simulink library "netZeroSpoolingControllerEllipsePath"  (R2020a)
settings: Solver=VariableStepAuto  StartTime=0.0  StopTime=10.0  RelTol=1e-3
undefined symbols (not defined in the file or in its folder): fltCtrl
libraries: runningAvg_ul x2, simulink x2, dspsigops x1
settings Model: Creator=jcreed2  LastModifiedBy=Josh Gaming
settings DataIOCC: ReturnWorkspaceOutputs=off
settings DebuggingCC: ArithmeticOperatorsInVariantConditions=warning
settings SFSimCC: CustomCodeUndefinedFunction=UseInterfaceOnly

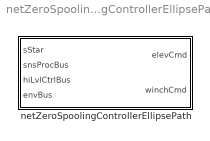
== system netZeroSpoolingControllerEllipsePath ==
  netZeroSpoolingControllerEllipsePath : Subsystem  mask{reelInDefl=23, reelOutDefl=0, sigmaVecInit=0, firstSpoolLap=fltCtrl.firstSpoolLap.Value}
      mask prompts: reelInDefl "Reel In Elevator Deflection [deg]"; reelOutDefl "Reel Out Elevator Deflection [deg]"; sigmaVecInit "Init Spooling Param Vec"; firstSpoolLap "First Lap to Start Spooling"

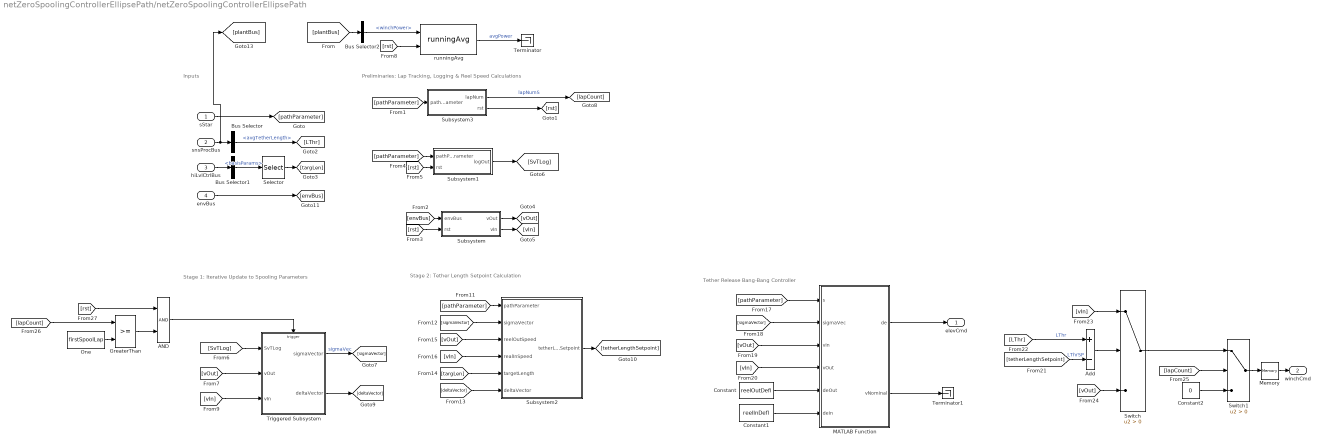
== system netZeroSpoolingControllerEllipsePath/netZeroSpoolingControllerEllipsePath ==
  note: Inputs
  note: Preliminaries: Lap Tracking, Logging & Reel Speed Calculations
  note: Stage 1: Iterative Update to Spooling Parameters
  note: Stage 2: Tether Length Setpoint Calculation
  note: Tether Release Bang-Bang Controller
  "sStar " : Inport
  snsProcBus : Inport  Port=2  OutDataTypeStr=Bus: sensorsProcessingBus
  hiLvlCtrlBus : Inport  Port=3  OutDataTypeStr=Bus: hiLvlCtrlBus
  envBus : Inport  Port=4  OutDataTypeStr=Bus: envBus
  AND : Logic  AllPortsSameDT=off  OutDataTypeStr=boolean
  Add : Sum  Inputs=+-
  Bus Selector : BusSelector  OutputSignals=avgTetherLength
  Bus Selector1 : BusSelector  OutputSignals=basisParams
  Bus Selector2 : BusSelector  OutputSignals=winchPower
  Constant : Constant  Value=reelOutDefl
  Constant1 : Constant  Value=reelInDefl
  Constant2 : Constant  Value=0
  GreaterThan : RelationalOperator  OutDataTypeStr=boolean  RndMeth=Simplest
  MATLAB Function : MATLAB Function  TreatAsAtomicUnit=on
  Memory : Memory
  One : Constant  Value=firstSpoolLap  OutDataTypeStr=Inherit: Inherit via back propagation
  Selector : Selector  InputPortWidth=5  IndexOptions=Index vector (dialog)  Indices=5  OutputSizes=1
  Subsystem : Subsystem
  Subsystem1 : Subsystem
  Subsystem2 : Subsystem
  Subsystem3 : Subsystem
  Switch : Switch  Criteria=u2 > Threshold
  Switch1 : Switch  Criteria=u2 > Threshold
  Terminator : Terminator
  Terminator1 : Terminator
  Triggered Subsystem : Subsystem  TreatAsAtomicUnit=on
  runningAvg : runningAvg_ul/runningAvg  SystemSampleTime=-1  Latency=0  AutoFrameSizeCalculation=off
  "elevCmd " : Outport  VectorParamsAs1DForOutWhenUnconnected=off
  winchCmd : Outport  Port=2  VectorParamsAs1DForOutWhenUnconnected=off
  wires:
  Switch/1 -> Switch1/1
  Constant/1 -> MATLAB Function/5(deOut)
  [rst] -> runningAvg/2
  [sigmaVector] -> MATLAB Function/2(sigmaVec)
  [lapCount] -> Switch1/2
  [vIn] -> Subsystem2/4(realInSpeed)
  runningAvg/1 -> Terminator/1  "avgPower"
  [rst] -> Subsystem1/2(rst)
  [SvTLog] -> Triggered Subsystem/1(SvTLog)
  "sStar "/1 -> [pathParameter]
  envBus/1 -> [envBus]
  Bus Selector1/1 -> Selector/1  "<basisParams>"
  [LThr] -> Add/1  "LThr"
  [pathParameter] -> Subsystem3/1(pathParameter)
  Bus Selector/1 -> [LThr]  "<avgTetherLength>"
  Add/1 -> Switch/2
  MATLAB Function/1(de) -> "elevCmd "/1
  Subsystem3/1(lapNum) -> [lapCount]  "lapNumS"
  [tetherLengthSetpoint] -> Add/2  "LThrSP"
  Constant1/1 -> MATLAB Function/6(deIn)
  Subsystem/2(vIn) -> [vIn]
  Constant2/1 -> Switch1/3
  [vOut] -> MATLAB Function/3(vIn)
  snsProcBus/1 -> [plantBus], Bus Selector/1
  Selector/1 -> [targLen]
  hiLvlCtrlBus/1 -> Bus Selector1/1
  [rst] -> Subsystem/2(rst)
  [vOut] -> Triggered Subsystem/2(vOut)
  Subsystem/1(vOut) -> [vOut]
  Triggered Subsystem/1("sigmaVector ") -> [sigmaVector]  "sigmaVec"
  [sigmaVector] -> Subsystem2/2(sigmaVector)
  [vIn] -> MATLAB Function/4(vOut)
  [deltaVector] -> Subsystem2/6(deltaVector)
  Subsystem3/2(rst) -> [rst]
  MATLAB Function/2(vNominal) -> Terminator1/1
  [vOut] -> Subsystem2/3(reelOutSpeed)
  [vIn] -> Switch/1
  [vIn] -> Triggered Subsystem/3(vIn)
  [pathParameter] -> MATLAB Function/1(s)
  Switch1/1 -> Memory/1
  [pathParameter] -> Subsystem2/1(pathParameter)
  [plantBus] -> Bus Selector2/1
  [targLen] -> Subsystem2/5(targetLength)
  [vOut] -> Switch/3
  Bus Selector2/1 -> runningAvg/1  "<winchPower>"
  [pathParameter] -> Subsystem1/1(pathParameter)
  [envBus] -> Subsystem/1(envBus)
  Triggered Subsystem/2(deltaVector) -> [deltaVector]
  Subsystem1/1(logOut) -> [SvTLog]
  GreaterThan/1 -> AND/2
  One/1 -> GreaterThan/2
  AND/1 -> Triggered Subsystem/Trigger
  [rst] -> AND/1
  [lapCount] -> GreaterThan/1
  Subsystem2/1(tetherLengthSetpoint) -> [tetherLengthSetpoint]
  Memory/1 -> winchCmd/1

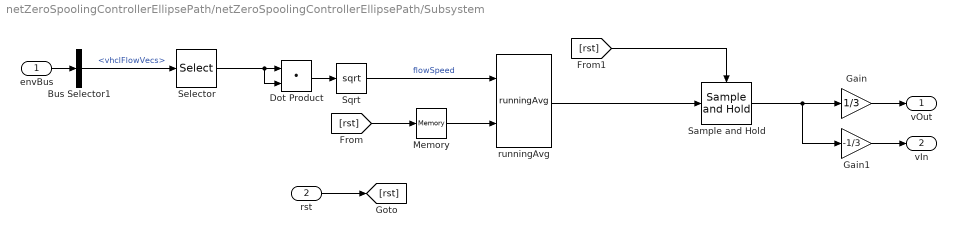
== system netZeroSpoolingControllerEllipsePath/netZeroSpoolingControllerEllipsePath/Subsystem ==
  envBus : Inport
  rst : Inport  Port=2
  Bus Selector1 : BusSelector  OutputSignals=vhclFlowVecs
  Dot Product : DotProduct  InputSameDT=on  OutDataTypeStr=Inherit: Inherit via internal rule
  Gain : Gain  Gain=1/3
  Gain1 : Gain  Gain=-1/3
  Memory : Memory
  Sample and Hold : dspsigops/Sample and Hold  trig=Rising edge  initCond=0  latchinput=off
  Selector : Selector  NumberOfDimensions=2  InputPortWidth=3  IndexOptions=Select all,Index vector (dialog)  Indices=[1 3],5  OutputSizes=1,1
  Sqrt : Sqrt  SaturateOnIntegerOverflow=on
  runningAvg : runningAvg_ul/runningAvg  SystemSampleTime=-1  Latency=0  AutoFrameSizeCalculation=off
  vOut : Outport  VectorParamsAs1DForOutWhenUnconnected=off
  vIn : Outport  Port=2  VectorParamsAs1DForOutWhenUnconnected=off
  wires:
  Dot Product/1 -> Sqrt/1
  Sample and Hold/1 -> Gain/1, Gain1/1
  Selector/1 -> Dot Product/1, Dot Product/2
  Sqrt/1 -> runningAvg/1  "flowSpeed"
  envBus/1 -> Bus Selector1/1
  rst/1 -> [rst]
  Gain1/1 -> vIn/1
  Bus Selector1/1 -> Selector/1  "<vhclFlowVecs>"
  Gain/1 -> vOut/1
  [rst] -> Memory/1
  runningAvg/1 -> Sample and Hold/1
  [rst] -> Sample and Hold/Trigger
  Memory/1 -> runningAvg/2

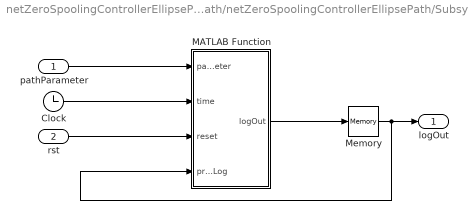
== system netZeroSpoolingControllerEllipsePath/netZeroSpoolingControllerEllipsePath/Subsystem1 ==
  pathParameter : Inport
  rst : Inport  Port=2
  Clock : Clock
  MATLAB Function : MATLAB Function  TreatAsAtomicUnit=on
  Memory : Memory  InitialCondition=zeros(1000,2)  InheritSampleTime=on
  logOut : Outport  VectorParamsAs1DForOutWhenUnconnected=off
  wires:
  pathParameter/1 -> MATLAB Function/1(pathParameter)
  Clock/1 -> MATLAB Function/2(time)
  rst/1 -> MATLAB Function/3(reset)
  MATLAB Function/1(logOut) -> Memory/1
  Memory/1 -> MATLAB Function/4(previousLog), logOut/1

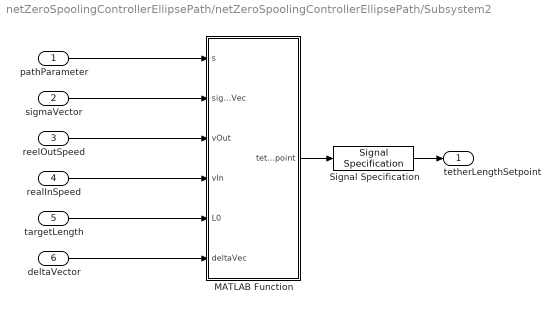
== system netZeroSpoolingControllerEllipsePath/netZeroSpoolingControllerEllipsePath/Subsystem2 ==
  pathParameter : Inport
  sigmaVector : Inport  Port=2
  reelOutSpeed : Inport  Port=3
  realInSpeed : Inport  Port=4
  targetLength : Inport  Port=5
  deltaVector : Inport  Port=6
  MATLAB Function : MATLAB Function  TreatAsAtomicUnit=on
  Signal Specification : SignalSpecification  Dimensions=[1 1]
  tetherLengthSetpoint : Outport  VectorParamsAs1DForOutWhenUnconnected=off
  wires:
  MATLAB Function/1(tetherLengthSetpoint) -> Signal Specification/1
  Signal Specification/1 -> tetherLengthSetpoint/1
  pathParameter/1 -> MATLAB Function/1(s)
  sigmaVector/1 -> MATLAB Function/2(sigmaVec)
  reelOutSpeed/1 -> MATLAB Function/3(vOut)
  realInSpeed/1 -> MATLAB Function/4(vIn)
  targetLength/1 -> MATLAB Function/5(L0)
  deltaVector/1 -> MATLAB Function/6(deltaVec)

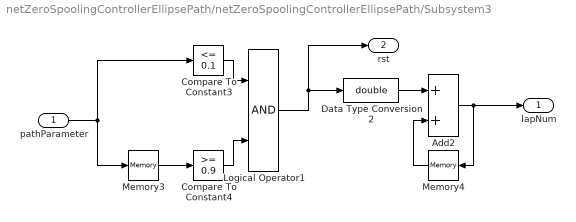
== system netZeroSpoolingControllerEllipsePath/netZeroSpoolingControllerEllipsePath/Subsystem3 ==
  pathParameter : Inport
  Add2 : Sum
  Compare To Constant3 : simulink/Logic and Bit Operations/Compare To Constant  relop=<=  const=0.1  OutDataTypeStr=boolean
  Compare To Constant4 : simulink/Logic and Bit Operations/Compare To Constant  relop=>=  const=0.9  OutDataTypeStr=boolean
  Data Type Conversion2 : DataTypeConversion  OutDataTypeStr=double
  Logical Operator1 : Logic  AllPortsSameDT=off  OutDataTypeStr=boolean
  Memory3 : Memory
  Memory4 : Memory
  lapNum : Outport  VectorParamsAs1DForOutWhenUnconnected=off
  rst : Outport  Port=2  VectorParamsAs1DForOutWhenUnconnected=off
  wires:
  Compare To Constant3/1 -> Logical Operator1/1
  Memory4/1 -> Add2/2
  Data Type Conversion2/1 -> Add2/1
  Add2/1 -> Memory4/1, lapNum/1
  Memory3/1 -> Compare To Constant4/1
  Compare To Constant4/1 -> Logical Operator1/2
  Logical Operator1/1 -> Data Type Conversion2/1, rst/1
  pathParameter/1 -> Memory3/1, Compare To Constant3/1

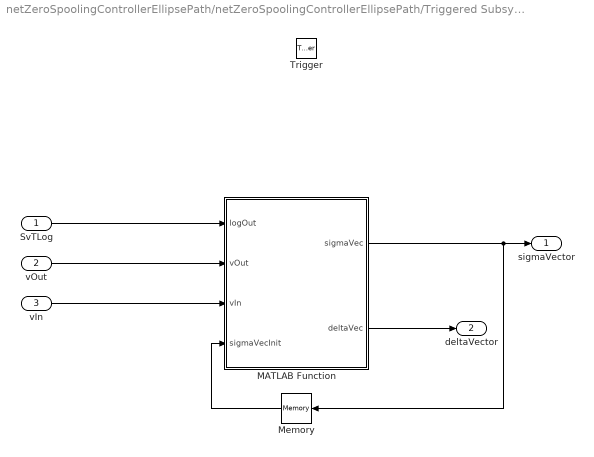
== system netZeroSpoolingControllerEllipsePath/netZeroSpoolingControllerEllipsePath/Triggered Subsystem ==
  SvTLog : Inport
  vOut : Inport  Port=2
  vIn : Inport  Port=3
  Trigger : TriggerPort  VariantControl=Variant
  MATLAB Function : MATLAB Function  TreatAsAtomicUnit=on
  Memory : Memory  InitialCondition=sigmaVecInit  InheritSampleTime=on
  "sigmaVector " : Outport  VectorParamsAs1DForOutWhenUnconnected=off
  deltaVector : Outport  Port=2  VectorParamsAs1DForOutWhenUnconnected=off
  wires:
  vOut/1 -> MATLAB Function/2(vOut)
  SvTLog/1 -> MATLAB Function/1(logOut)
  vIn/1 -> MATLAB Function/3(vIn)
  MATLAB Function/1(sigmaVec) -> Memory/1, "sigmaVector "/1
  MATLAB Function/2(deltaVec) -> deltaVector/1
  Memory/1 -> MATLAB Function/4(sigmaVecInit)

== matlab function netZeroSpoolingControllerEllipsePath/Triggered Subsystem/MATLAB Function ==
  data: logOut input; sigmaVec output; vOut input; vIn input; sigmaVecInit input; deltaVec output
function [sigmaVec, deltaVec] = fcn(logOut,vOut,vIn, sigmaVecInit)
sc = sigmaVecInit(1);
sw = sigmaVecInit(2);
sigmaVec = sigmaVecInit;

cleanLog = [ 0 0; ...
    logOut(and(and(logOut(:,1)~=0,logOut(:,2)~=0),and(~isnan(logOut(:,1)),~isnan(logOut(:,2)))),:)];
 
% Extract regions
r1 = cleanLog(and(cleanLog(:,1)>=0        ,cleanLog(:,1)<sc-sw),:);
r2 = cleanLog(and(cleanLog(:,1)>=sc-sw    ,cleanLog(:,1)<sc+sw),:);
r3 = cleanLog(and(cleanLog(:,1)>=sc+sw    ,cleanLog(:,1)<0.5+sc-sw),:);
r4 = cleanLog(and(cleanLog(:,1)>=0.5+sc-sw,cleanLog(:,1)<0.5+sc+sw),:);
r5 = cleanLog(and(cleanLog(:,1)>=0.5+sc+sw,cleanLog(:,1)<=1),:);

% Calculate average numerical derivative in each region ds/dt
ds1 = mean(diff(r1(:,1))./diff(r1(:,2)));
ds2 = mean(diff(r2(:,1))./diff(r2(:,2)));
ds3 = mean(diff(r3(:,1))./diff(r3(:,2)));
ds4 = mean(diff(r4(:,1))./diff(r4(:,2)));
ds5 = mean(diff(r5(:,1))./diff(r5(:,2)));

deltaVec = [ds1 ds2 ds3 ds4 ds5]';

dsInv = diag([1/ds1 1/ds2 1/ds3 1/ds4 1/ds5]);

V = diag([vOut vIn vOut vIn vOut]);

Delta = eye(5);
Delta(2,1) = -1;
Delta(3,2) = -1;
Delta(4,3) = -1;
Delta(5,4) = -1;

A  = [ 0  0 0.5 0.5 1]';
B1 = [ 1  1   1   1 0]';
B2 = [-1  1  -1   1 0]';

c1 = ones(1,5)*V*dsInv*Delta*(A+B1*sc);
c2 = ones(1,5)*V*dsInv*Delta*B2;
if ~any(isnan([c1 c2]))
    sw = min([max([-c1/c2 0]) sc]); % 0<=sw<=sc
end
sigmaVec(2) = sw;

== matlab function netZeroSpoolingControllerEllipsePath/Subsystem1/MATLAB Function ==
  data: pathParameter input; logOut output; time input; reset input; previousLog input
function logOut = fcn(pathParameter,time , reset,previousLog)

if reset 
    previousLog = nan(1000,2);
end

logOut = previousLog; 

index = min([max([round(pathParameter*1000),1]),1000]);
logOut(index,1) = pathParameter;
logOut(index,2) = time;
end

== matlab function netZeroSpoolingControllerEllipsePath/Subsystem2/MATLAB Function ==
  data: s input; tetherLengthSetpoint output size=[1 1]; sigmaVec input; vOut input; vIn input; L0 input; deltaVec input
function tetherLengthSetpoint = fcn(s,sigmaVec,vOut,vIn,L0,deltaVec)

tetherLengthSetpoint = LThrInt1(s,sigmaVec,vOut,vIn,L0,deltaVec);
end

== matlab function netZeroSpoolingControllerEllipsePath/MATLAB Function ==
  data: s input; de output; sigmaVec input; vIn input; vOut input; deOut input; deIn input; vNominal output
function [de,vNominal] = fcn(s,sigmaVec, vIn, vOut, deOut, deIn)

vNominal = vOut;
de = deOut;

sc = sigmaVec(1);
sw = sigmaVec(2);

if s>=sc-sw && s<=sc+sw
    vNominal = vIn;
    de = deIn;
    return
end

if s>=0.5+sc-sw && s<=0.5+sc+sw
    vNominal = vIn;
    de = deIn;
    return
end
end
